simulink model "SF035A_DampgPahFwl"  (R2013b)
settings: Solver=FixedStepDiscrete  SolverMode=SingleTasking  StartTime=0.0  StopTime=1  FixedStep=0.002  RelTol=1e-3
undefined symbols (not defined in the file): ARCHGLBPRM_2MILLISEC_SEC_F32, DampgPahFwlDampgCmdFwlOverLimDiagcFailStep, DampgPahFwlDampgCmdFwlOverLimDiagcPassStep, DampgPahFwlInertiaCmpCmdFwlOverLimDiagcFailStep, DampgPahFwlInertiaCmpCmdFwlOverLimDiagcPassStep, DMPGCMDREACHED_CNT_U08, MfgEnaSt1, NtcNr1, NtcSts1, sigbuilder_block, SigQlfr1, VBICCMDREACHED_CNT_U08
libraries: simulink x23, Fil x12, FixdToFloat x7, FloatToFixd x5, BilnrIntrpnCmnX x4, LnrIntrpn x3, NxtrLim x3, NxtrAbslt x2, NxtrSign x2, NxtrMax x1
(part 1 of 3)
settings Model: Creator=HariP  LastModifiedBy=SNEHAP1
settings SolverCC: AutoInsertRateTranBlk=on  InsertRTBMode=Always
settings DataIOCC: LimitDataPoints=off  SaveFormat=Structure  ReturnWorkspaceOutputs=on
settings OptimizationCC: BlockReduction=off  InlineParams=on  ZeroExternalMemoryAtStartup=off  ZeroInternalMemoryAtStartup=off  OptimizeModelRefInitCode=on  LifeSpan=1
settings DebuggingCC: SignalInfNanChecking=error  SignalRangeChecking=warning  UnderspecifiedInitializationDetection=Simplified  SolverPrmCheckMsg=error  InheritedTsInSrcMsg=error  DiscreteInheritContinuousMsg=error  SingleTaskRateTransMsg=error  TasksWithSamePriorityMsg=error  SigSpecEnsureSampleTimeMsg=error  CheckMatrixSingularityMsg=error  ParameterUnderflowMsg=error  ParameterPrecisionLossMsg=error  ParameterTunabilityLossMsg=error  FixptConstUnderflowMsg=warning  FixptConstOverflowMsg=warning  VectorMatrixConversionMsg=error  SignalLabelMismatchMsg=error  UnconnectedInputMsg=error  UnconnectedOutputMsg=error  UnconnectedLineMsg=error  SFcnCompatibilityMsg=error  UniqueDataStoreMsg=warning  BusObjectLabelMismatch=error  RootOutportRequireBusObject=error  AssertControl=DisableAll  ModelReferenceIOMsg=error  ModelReferenceVersionMismatchMessage=warning  ModelReferenceIOMismatchMessage=error  ModelReferenceCSMismatchMessage=warning  ModelReferenceDataLoggingMessage=error  StateNameClashWarn=warning  StrictBusMsg=ErrorOnBusTreatedAsVector  NonBusSignalsTreatedAsBus=error  SFUnexpectedBacktrackingDiag=error  SFInvalidInputDataAccessInChartInitDiag=error  SFNoUnconditionalDefaultTransitionDiag=error  SFTransitionOutsideNaturalParentDiag=error  SFUnconditionalTransitionShadowingDiag=error  SFUndirectedBroadcastEventsDiag=error
settings ModelReferenceCC: ModelReferenceNumInstancesAllowed=Single
settings RTWCC: SystemTargetFile=autosar.tlc  GenCodeOnly=on  TemplateMakefile=ert_default_tmf  Description=AUTOSAR  GenerateReport=on  ProcessScript=autosar_make_rtw_hook  LaunchReport=on
settings CodeAppCC: GenerateComments=off  IgnoreCustomStorageClasses=off  CustomSymbolStrType=$N$R$M  CustomSymbolStrBlkIO=$N$M  SimulinkBlockComments=off
settings STFCustomTargetCC: ParMdlRefBuildCompliant=on  CompOptLevelCompliant=on  IncludeMdlTerminateFcn=off  CombineOutputUpdateFcns=on  SuppressErrorStatus=on  ERTFirstTimeCompliant=on  ERTCustomFileBanners=on  SupportNonFinite=off  SupportComplex=off  SupportContinuousTime=off  SupportNonInlinedSFcns=off  MATLABClassNameForMDSCustomization=Simulink.SoftwareTarget.ERTCustomization  AutosarCompliant=on  GRTInterface=off  SystemTargetFile=autosar.tlc
settings ERTTargetCC: CodeReplacementLibrary=ANSI_C  ConcurrentExecutionCompliant=off  IncludeMdlTerminateFcn=off  SuppressErrorStatus=on  SupportNonFinite=off  SupportComplex=off  ModelStepFunctionPrototypeControlCompliant=off  CPPClassGenCompliant=off  AutosarCompliant=on  InlinedParameterPlacement=NonHierarchical  ERTCustomFileTemplate=example_file_process.tlc  EnableUserReplacementTypes=on

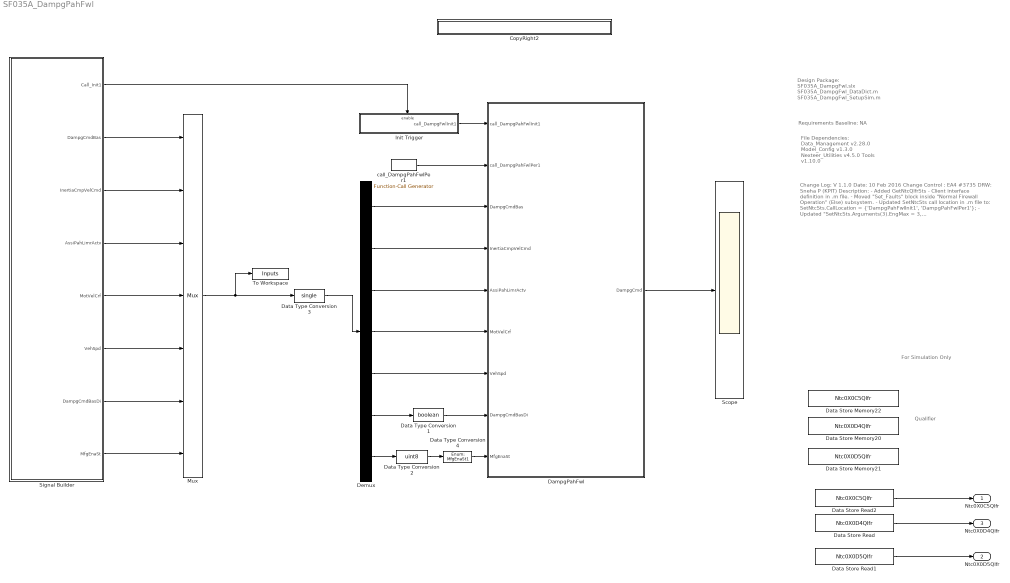
== system SF035A_DampgPahFwl ==
  note: Qualifier
  note: For Simulation Only
  note: Requirements Baseline: NA
  note: Design Package:
      | SF035A_DampgFwl.slx
      | SF035A_DampgFwl_DataDict.m
      | SF035A_DampgFwl_SetupSim.m
  note: File Dependencies:
      | Data_Management v2.28.0
      | Model_Config v1.3.0
      | Nexteer_Utilities v4.5.0
      | Tools v1.10.0
  note: Change Log:  V 1.1.0
      | Date: 10 Feb 2016
      | Change Control :  EA4 #3735
      | DRW: Sneha P (KPIT)
      | Description:
      | - Added GetNtcQlfrSts - Client interface definition in .m file.
      | - Moved "Set_Faults" block inside "Normal Firewall Operation"
      |   (Else) subsystem.
      | - Updated SetNtcSts call location in .m file to:
      |   SetNtcSts.CallLocation = {'DampgPahFwlInit1', 'DampgPahFwlPer1'};
      | - Updated "SetNtcSts.Arguments(3).EngMax = 3,
      |   SetNtcSts.Arguments(3).EngDT = enum.NtcSts1;,
      |   SetNtcSts.Arguments(3).Units = 'Cnt' in .m file.
      |
      |
      | Change Log:  V 1.0.0
      | Date: 01 Feb 2016
      | Change Control #:  EA4 #3606
      | DRW: Hari Prasad / Muragesh Asundi (KPIT)
      | Description:
      | - Initial Release of EA4 V1.0.0 from EA3 V12.0.X
  CopyRight2 : Subsystem  Description=|  mask(Copyright Information){none=on}
      | Copyright info block.                                               
      |                                                                     
      | Place copyright information at the top of every subsystem in design.
      mask prompts: none "No parameters"
      mask help: Place copyright information at the top of every subsystem in design.
      mask Display:
      | NxtrConf = 'Nexteer Confidential';
      | 
      | sys = bdroot; %handle for the current model ("system")
      | first = get_param(sys,'Created');
      | first = first(end-3:end);  %year is last four digits
      | 
      | last = get_param(sys,'LastModifiedDate');
      | if isempty(last)
      |     last = datestr(now,'yyyy');
      | else
      |     last = last(end-3:end);
      | end
      | 
      | if strcmp(first,last)
      |     fprintf('%s -- Copyright %s Nexteer',NxtrConf,first)
      | else
      |     fprintf('%s -- %s%s- %s Nexteer',NxtrConf,char(169),first,last)
      | end
  DampgPahFwl : Subsystem
  Data Store Memory20 : DataStoreMemory  DataStoreName=Ntc0X0D4Qlfr  InitialValue=SigQlfr1.SIGQLFR_NORES  OutDataTypeStr=Enum: SigQlfr1
  Data Store Memory21 : DataStoreMemory  DataStoreName=Ntc0X0D5Qlfr  InitialValue=SigQlfr1.SIGQLFR_NORES  OutDataTypeStr=Enum: SigQlfr1
  Data Store Memory22 : DataStoreMemory  DataStoreName=Ntc0X0C5Qlfr  InitialValue=SigQlfr1.SIGQLFR_NORES  OutDataTypeStr=Enum: SigQlfr1
  Data Store Read : DataStoreRead  DataStoreName=Ntc0X0D4Qlfr  SampleTime=0.002
  Data Store Read1 : DataStoreRead  DataStoreName=Ntc0X0D5Qlfr  SampleTime=0.002
  Data Store Read2 : DataStoreRead  DataStoreName=Ntc0X0C5Qlfr  SampleTime=0.002
  Data Type Conversion1 : DataTypeConversion  OutDataTypeStr=boolean
  Data Type Conversion2 : DataTypeConversion  OutDataTypeStr=uint8
  Data Type Conversion3 : DataTypeConversion  OutDataTypeStr=single
  Data Type Conversion4 : DataTypeConversion  OutDataTypeStr=Enum: MfgEnaSt1
  Demux : Demux  Outputs=7
  Init Trigger : Subsystem  TreatAsAtomicUnit=on
  Mux : Mux  Inputs=7
  Scope : Scope
  Signal Builder : Subsystem  Tag=STV Subsys  LoadFcn=sigbuilder_block('load');  StartFcn=sigbuilder_block('start');  StopFcn=sigbuilder_block('stop');  ClipboardFcn=sigbuilder_block('clipboard');  mask(Sigbuilder block){}
      mask help: Simulink:masks:SigbuilderBlock_MD
      mask init:
      | if ~strcmp(get_param(bdroot(gcbh),'SimulationStatus'),'stopped') tuvar = sigbuilder_block('maskInit'); end
      settings: CopyFcn=sigbuilder_block('copy');  DeleteFcn=sigbuilder_block('delete');  ModelCloseFcn=sigbuilder_block('modelClose');  PreSaveFcn=sigbuilder_block('preSave');  PauseFcn=sigbuilder_block('pause');  ContinueFcn=sigbuilder_block('continue');  NameChangeFcn=sigbuilder_block('namechange');  OpenFcn=sigbuilder_block('open',[0 30 1024.5 489 ]);  CloseFcn=sigbuilder_block('close');
      mask Display: plot(0, 0, 100, 100,[2, 2, 32, 32, 2], [68, 8, 8, 68, 68],[32, 2], [38, 38], [32, 19, 2],[53, 60, 44], [32, 17, 17, 2],[16, 16, 31, 31]);txt = getActiveGroup(gcbh);text(2, 100, txt,'verticalAlignment', 'top');
  To Workspace : ToWorkspace  VariableName=Inputs  SampleTime=-1
  call_DampgPahFwlPer1 : simulink/Ports & Subsystems/Function-Call Generator  RequirementInfo={} %GIDa_4a149a05_295f_452b_ba1c_52fd600be539  sample_time=0.002  numberOfIterations=1
  Ntc0X0C5Qlfr : Outport
  Ntc0X0D5Qlfr : Outport  Port=2
  Ntc0X0D4Qlfr : Outport  Port=3
  wires:
  DampgPahFwl/1(DampgCmd) -> Scope/1
  Init Trigger/1(call_DampgFwlInit1) -> DampgPahFwl/1(call_DampgPahFwlInit1)
  call_DampgPahFwlPer1/1 -> DampgPahFwl/2(call_DampgPahFwlPer1)
  Data Store Read/1 -> Ntc0X0D4Qlfr/1
  Data Store Read1/1 -> Ntc0X0D5Qlfr/1
  Data Store Read2/1 -> Ntc0X0C5Qlfr/1
  Mux/1 -> To Workspace/1, Data Type Conversion3/1
  Data Type Conversion3/1 -> Demux/1
  Demux/4 -> DampgPahFwl/6(MotVelCrf)
  Demux/2 -> DampgPahFwl/4(InertiaCmpVelCmd)
  Demux/5 -> DampgPahFwl/7(VehSpd)
  Demux/1 -> DampgPahFwl/3(DampgCmdBas)
  Demux/6 -> Data Type Conversion1/1
  Demux/7 -> Data Type Conversion2/1
  Signal Builder/1(Call_Init1) -> Init Trigger/Enable
  Signal Builder/4(AssiPahLimrActv) -> Mux/3
  Signal Builder/5(MotVelCrf) -> Mux/4
  Signal Builder/3(InertiaCmpVelCmd) -> Mux/2
  Signal Builder/6(VehSpd) -> Mux/5
  Signal Builder/2(DampgCmdBas) -> Mux/1
  Signal Builder/7(DampgCmdBasDi) -> Mux/6
  Signal Builder/8(MfgEnaSt) -> Mux/7
  Data Type Conversion1/1 -> DampgPahFwl/8(DampgCmdBasDi)
  Demux/3 -> DampgPahFwl/5(AssiPahLimrActv)
  Data Type Conversion2/1 -> Data Type Conversion4/1
  Data Type Conversion4/1 -> DampgPahFwl/9(MfgEnaSt)

== system SF035A_DampgPahFwl/CopyRight2 ==

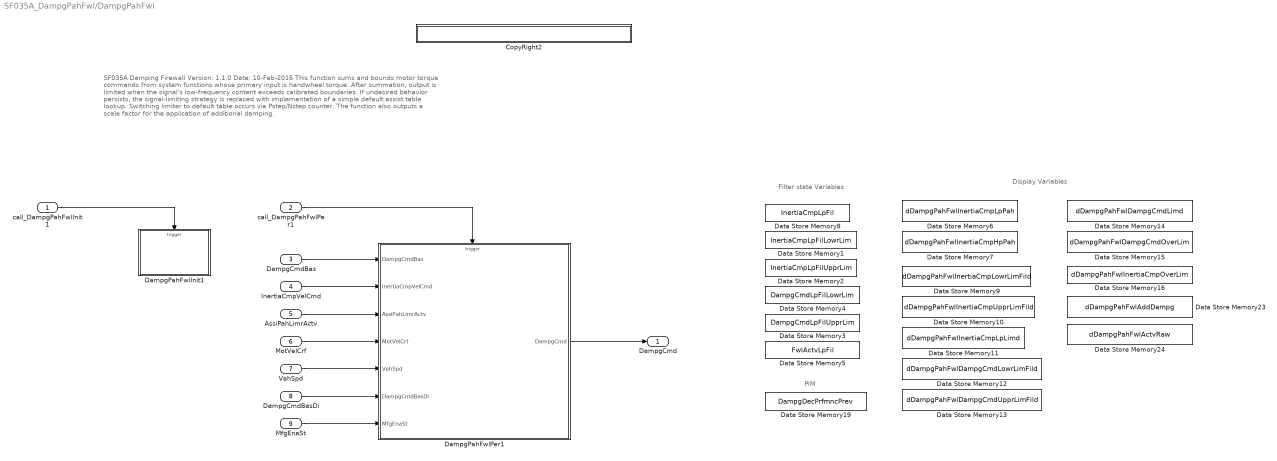
== system SF035A_DampgPahFwl/DampgPahFwl ==
  note: PIM
  note: Filter state Variables
  note: Display Variables
  note: SF035A Damping Firewall
      | Version: 1.1.0      Date: 10-Feb-2016
      |
      | This function sums and bounds motor torque commands from system functions whose primary input is handwheel torque.  After summation, output is limited when the signal's low-frequency content
      | exceeds calibrated boundaries.  If undesired behavior persists,  the signal-limiting strategy is replaced with implementation of a simple default assist table lookup.  Switching limiter to default table
      | occurs via Pstep/Nstep counter.  The function also outputs a scale factor for the application of additional damping.
  call_DampgPahFwlInit1 : Inport
  call_DampgPahFwlPer1 : Inport  Port=2
  DampgCmdBas : Inport  Port=3
  InertiaCmpVelCmd : Inport  Port=4
  AssiPahLimrActv : Inport  Port=5
  MotVelCrf : Inport  Port=6
  VehSpd : Inport  Port=7
  DampgCmdBasDi : Inport  Port=8
  MfgEnaSt : Inport  Port=9
  CopyRight2 : Subsystem  Description=|  mask(Copyright Information){none=on}
      | Copyright info block.                                               
      |                                                                     
      | Place copyright information at the top of every subsystem in design.
      mask prompts: none "No parameters"
      mask help: Place copyright information at the top of every subsystem in design.
      mask Display:
      | NxtrConf = 'Nexteer Confidential';
      | 
      | sys = bdroot; %handle for the current model ("system")
      | first = get_param(sys,'Created');
      | first = first(end-3:end);  %year is last four digits
      | 
      | last = get_param(sys,'LastModifiedDate');
      | if isempty(last)
      |     last = datestr(now,'yyyy');
      | else
      |     last = last(end-3:end);
      | end
      | 
      | if strcmp(first,last)
      |     fprintf('%s -- Copyright %s Nexteer',NxtrConf,first)
      | else
      |     fprintf('%s -- %s%s- %s Nexteer',NxtrConf,char(169),first,last)
      | end
  DampgPahFwlInit1 : Subsystem  TreatAsAtomicUnit=on
  DampgPahFwlPer1 : Subsystem
  Data Store Memory1 : DataStoreMemory  DataStoreName=InertiaCmpLpFilLowrLim  InitialValue=struct('FilSt',single(0),'FilGain',single(0))  OutDataTypeStr=Bus: FilLpRec1  StateMustResolveToSignalObject=on
  Data Store Memory10 : DataStoreMemory  DataStoreName=dDampgPahFwlInertiaCmpUpprLimFild  StateMustResolveToSignalObject=on
  Data Store Memory11 : DataStoreMemory  DataStoreName=dDampgPahFwlInertiaCmpLpLimd  InitialValue=[]  StateMustResolveToSignalObject=on
  Data Store Memory12 : DataStoreMemory  DataStoreName=dDampgPahFwlDampgCmdLowrLimFild  InitialValue=[]  StateMustResolveToSignalObject=on
  Data Store Memory13 : DataStoreMemory  DataStoreName=dDampgPahFwlDampgCmdUpprLimFild  InitialValue=[]  StateMustResolveToSignalObject=on
  Data Store Memory14 : DataStoreMemory  DataStoreName=dDampgPahFwlDampgCmdLimd  InitialValue=[]  StateMustResolveToSignalObject=on
  Data Store Memory15 : DataStoreMemory  DataStoreName=dDampgPahFwlDampgCmdOverLim  InitialValue=[]  StateMustResolveToSignalObject=on
  Data Store Memory16 : DataStoreMemory  DataStoreName=dDampgPahFwlInertiaCmpOverLim  InitialValue=[]  StateMustResolveToSignalObject=on
  Data Store Memory19 : DataStoreMemory  DataStoreName=DampgDecPrfmncPrev  StateMustResolveToSignalObject=on
  Data Store Memory2 : DataStoreMemory  DataStoreName=InertiaCmpLpFilUpprLim  InitialValue=struct('FilSt',single(0),'FilGain',single(0))  OutDataTypeStr=Bus: FilLpRec1  StateMustResolveToSignalObject=on
  Data Store Memory23 : DataStoreMemory  DataStoreName=dDampgPahFwlAddDampg  InitialValue=[]  StateMustResolveToSignalObject=on
  Data Store Memory24 : DataStoreMemory  DataStoreName=dDampgPahFwlActvRaw  InitialValue=[]  StateMustResolveToSignalObject=on
  Data Store Memory3 : DataStoreMemory  DataStoreName=DampgCmdLpFilUpprLim  InitialValue=struct('FilSt',single(0),'FilGain',single(0))  OutDataTypeStr=Bus: FilLpRec1  StateMustResolveToSignalObject=on
  Data Store Memory4 : DataStoreMemory  DataStoreName=DampgCmdLpFilLowrLim  InitialValue=struct('FilSt',single(0),'FilGain',single(0))  OutDataTypeStr=Bus: FilLpRec1  StateMustResolveToSignalObject=on
  Data Store Memory5 : DataStoreMemory  DataStoreName=FwlActvLpFil  InitialValue=struct('FilSt',single(0),'FilGain',single(0))  OutDataTypeStr=Bus: FilLpRec1  StateMustResolveToSignalObject=on
  Data Store Memory6 : DataStoreMemory  DataStoreName=dDampgPahFwlInertiaCmpLpPah  InitialValue=[]  StateMustResolveToSignalObject=on
  Data Store Memory7 : DataStoreMemory  DataStoreName=dDampgPahFwlInertiaCmpHpPah  InitialValue=[]  StateMustResolveToSignalObject=on
  Data Store Memory8 : DataStoreMemory  DataStoreName=InertiaCmpLpFil  InitialValue=struct('FilSt',single(0),'FilGain',single(0))  OutDataTypeStr=Bus: FilLpRec1  StateMustResolveToSignalObject=on
  Data Store Memory9 : DataStoreMemory  DataStoreName=dDampgPahFwlInertiaCmpLowrLimFild  InitialValue=[]  StateMustResolveToSignalObject=on
  DampgCmd : Outport
  wires:
  DampgPahFwlPer1/1(DampgCmd) -> DampgCmd/1
  call_DampgPahFwlPer1/1 -> DampgPahFwlPer1/Trigger
  DampgCmdBas/1 -> DampgPahFwlPer1/1(DampgCmdBas)
  InertiaCmpVelCmd/1 -> DampgPahFwlPer1/2(InertiaCmpVelCmd)
  AssiPahLimrActv/1 -> DampgPahFwlPer1/3(AssiPahLimrActv)
  VehSpd/1 -> DampgPahFwlPer1/5(VehSpd)
  MotVelCrf/1 -> DampgPahFwlPer1/4(MotVelCrf)
  DampgCmdBasDi/1 -> DampgPahFwlPer1/6(DampgCmdBasDi)
  MfgEnaSt/1 -> DampgPahFwlPer1/7(MfgEnaSt)
  call_DampgPahFwlInit1/1 -> DampgPahFwlInit1/Trigger

== system SF035A_DampgPahFwl/Init Trigger ==
  Enable : EnablePort
  CopyRight2 : Subsystem  Description=|  mask(Copyright Information){none=on}
      | Copyright info block.                                               
      |                                                                     
      | Place copyright information at the top of every subsystem in design.
      mask prompts: none "No parameters"
      mask help: Place copyright information at the top of every subsystem in design.
      mask Display:
      | NxtrConf = 'Nexteer Confidential';
      | 
      | sys = bdroot; %handle for the current model ("system")
      | first = get_param(sys,'Created');
      | first = first(end-3:end);  %year is last four digits
      | 
      | last = get_param(sys,'LastModifiedDate');
      | if isempty(last)
      |     last = datestr(now,'yyyy');
      | else
      |     last = last(end-3:end);
      | end
      | 
      | if strcmp(first,last)
      |     fprintf('%s -- Copyright %s Nexteer',NxtrConf,first)
      | else
      |     fprintf('%s -- %s%s- %s Nexteer',NxtrConf,char(169),first,last)
      | end
  call_DampgPahFwlInit : simulink/Ports & Subsystems/Function-Call Generator  sample_time=0  numberOfIterations=1
  call_DampgFwlInit1 : Outport
  wires:
  call_DampgPahFwlInit/1 -> call_DampgFwlInit1/1

== system SF035A_DampgPahFwl/Signal Builder ==
  Demux : Demux  Tag=STV Demux  Outputs=8
  FromWs : FromWorkspace  Tag=STV FromWs  VariableName=tuvar  SampleTime=0
      SigBuilderData=|
      | common.afterFinalStr = 'Extrapolate'
      | common.sampleTime = 0
      | dataSet.timeRange = [0 0.31]
      | dataSet.name = 'TestCase_1'
      | sbobj.Name = 'Signal Builder'
      | sbobj.Groups.Name = 'TestCase_1'
      | sbobj.Groups.Signals(1).Name = 'Call_Init1'
      | sbobj.Groups.Signals(1).XData = [0 0.002 0.004 0.006 0.008 0.01 0.012 0.014 0.016 0.018 0.02 0.022 0.024 0.026 0.028 0.03 0.032 0.034 0.036 0.038 0.04 0.042 0.044 0.046 0.048 0.05 0.052 0.054 0.056 0.058 0.06 0.062 0.064 0.066 0.068 0.07 0.072 0.074 0.076 0.078 0.08 0.082 0.084 0.086 0.088 0.09 0.092 0.094 0.096 0.098 0.1 0.102 0.104 0.106 0.108 0.11 0.112 0.114 0.116 0.118 0.12 0.122 0.124 0.126 0.128 0.13 0.132 0.134 0.136 0.138 0.14 0.142 0.144 0.146 0.148 0.15 0.152 0.154 0.156 0.158 0.16 0.162 0.164 0.166 0.168 0.17 0.172 0.174 0.176 0.178 0.18 0.182 0.184 0.186 0.188 0.19 0.192 0.194 0.196 0.198 0.2 0.202 0.204 0.206 0.208 0.21 0.212 0.214 0.216 0.218 0.22 0.222 0.224 0.226 0.228 0.23 0.232 0.234 0.236 0.238 0.24 0.242 0.244 0.246 0.248 0.25 0.252 0.254 0.256 0.258 0.26 0.262 0.264 0.266 0.268 0.27 0.272 0.274 0.276 0.278 0.28 0.282 0.284 0.286 0.288 0.29 0.292 0.294 0.296 0.298 0.3 0.302 0.304 0.306 0.308 0.31]
      | sbobj.Groups.Signals(1).YData = [1 0 0 0 0 0 0 0 0 0 0 0 0 0 0 0 0 0 0 0 0 0 0 0 0 0 0 0 0 0 0 0 0 0 0 0 0 0 0 0 0 0 0 0 0 0 0 0 0 0 0 0 0 0 0 0 0 0 0 0 0 0 0 0 0 0 0 0 0 0 0 0 0 0 0 0 0 0 0 0 0 0 0 0 0 0 0 0 0 0 0 0 0 0 0 0 0 0 0 0 0 0 0 0 0 0 0 0 0 0 0 0 0 0 0 0 0 0 0 0 0 0 0 0 0 0 0 0 0 0 0 0 0 0 0 0 0 0 0 0 0 0 0 0 0 0 0 0 0 0 0 0 0 0 0 0]
      | sbobj.Groups.Signals(2).Name = 'DampgCmdBas'
      | sbobj.Groups.Signals(2).XData = [0 0.002 0.004 0.006 0.008 0.01 0.012 0.014 0.016 0.018 0.02 0.022 0.024 0.026 0.028 0.03 0.032 0.034 0.036 0.038 0.04 0.042 0.044 0.046 0.048 0.05 0.052 0.054 0.056 0.058 0.06 0.062 0.064 0.066 0.068 0.07 0.072 0.074 0.076 0.078 0.08 0.082 0.084 0.086 0.088 0.09 0.092 0.094 0.096 0.098 0.1 0.102 0.104 0.106 0.108 0.11 0.112 0.114 0.116 0.118 0.12 0.122 0.124 0.126 0.128 0.13 0.132 0.134 0.136 0.138 0.14 0.142 0.144 0.146 0.148 0.15 0.152 0.154 0.156 0.158 0.16 0.162 0.164 0.166 0.168 0.17 0.172 0.174 0.176 0.178 0.18 0.182 0.184 0.186 0.188 0.19 0.192 0.194 0.196 0.198 0.2 0.202 0.204 0.206 0.208 0.21 0.212 0.214 0.216 0.218 0.22 0.222 0.224 0.226 0.228 0.23 0.232 0.234 0.236 0.238 0.24 0.242 0.244 0.246 0.248 0.25 0.252 0.254 0.256 0.258 0.26 0.262 0.264 0.266 0.268 0.27 0.272 0.274 0.276 0.278 0.28 0.282 0.284 0.286 0.288 0.29 0.292 0.294 0.296 0.298 0.3 0.302 0.304 0.306 0.308 0.31]
      | sbobj.Groups.Signals(2).YData = [-8.8 -8.78263521017 -8.70559653007 -8.56749434528 -8.3692973434 -8.11239573398 -7.79859149723 -7.43008574442 -7.00946327861 -6.5396744642 -6.02401453217 -5.46610046645 ... (156 elements, 1x156)]
      | sbobj.Groups.Signals(3).Name = 'InertiaCmpVelCmd'
      | sbobj.Groups.Signals(3).XData = [0 0.002 0.004 0.006 0.008 0.01 0.012 0.014 0.016 0.018 0.02 0.022 0.024 0.026 0.028 0.03 0.032 0.034 0.036 0.038 0.04 0.042 0.044 0.046 0.048 0.05 0.052 0.054 0.056 0.058 0.06 0.062 0.064 0.066 0.068 0.07 0.072 0.074 0.076 0.078 0.08 0.082 0.084 0.086 0.088 0.09 0.092 0.094 0.096 0.098 0.1 0.102 0.104 0.106 0.108 0.11 0.112 0.114 0.116 0.118 0.12 0.122 0.124 0.126 0.128 0.13 0.132 0.134 0.136 0.138 0.14 0.142 0.144 0.146 0.148 0.15 0.152 0.154 0.156 0.158 0.16 0.162 0.164 0.166 0.168 0.17 0.172 0.174 0.176 0.178 0.18 0.182 0.184 0.186 0.188 0.19 0.192 0.194 0.196 0.198 0.2 0.202 0.204 0.206 0.208 0.21 0.212 0.214 0.216 0.218 0.22 0.222 0.224 0.226 0.228 0.23 0.232 0.234 0.236 0.238 0.24 0.242 0.244 0.246 0.248 0.25 0.252 0.254 0.256 0.258 0.26 0.262 0.264 0.266 0.268 0.27 0.272 0.274 0.276 0.278 0.28 0.282 0.284 0.286 0.288 0.29 0.292 0.294 0.296 0.298 0.3 0.302 0.304 0.306 0.308 0.31]
      | sbobj.Groups.Signals(3).YData = [0 0.736365021324 1.4675649711 2.18847100705 2.8940264913 3.57928245907 4.2394323321 4.86984563334 5.46610046645 6.02401453217 6.5396744642 7.00946327861 ... (156 elements, 1x156)]
      | sbobj.Groups.Signals(4).Name = 'AssiPahLimrActv'
      | sbobj.Groups.Signals(4).XData = [0 0.002 0.004 0.006 0.008 0.01 0.012 0.014 0.016 0.018 0.02 0.022 0.024 0.026 0.028 0.03 0.032 0.034 0.036 0.038 0.04 0.042 0.044 0.046 0.048 0.05 0.052 0.054 0.056 0.058 0.06 0.062 0.064 0.066 0.068 0.07 0.072 0.074 0.076 0.078 0.08 0.082 0.084 0.086 0.088 0.09 0.092 0.094 0.096 0.098 0.1 0.102 0.104 0.106 0.108 0.11 0.112 0.114 0.116 0.118 0.12 0.122 0.124 0.126 0.128 0.13 0.132 0.134 0.136 0.138 0.14 0.142 0.144 0.146 0.148 0.15 0.152 0.154 0.156 0.158 0.16 0.162 0.164 0.166 0.168 0.17 0.172 0.174 0.176 0.178 0.18 0.182 0.184 0.186 0.188 0.19 0.192 0.194 0.196 0.198 0.2 0.202 0.204 0.206 0.208 0.21 0.212 0.214 0.216 0.218 0.22 0.222 0.224 0.226 0.228 0.23 0.232 0.234 0.236 0.238 0.24 0.242 0.244 0.246 0.248 0.25 0.252 0.254 0.256 0.258 0.26 0.262 0.264 0.266 0.268 0.27 0.272 0.274 0.276 0.278 0.28 0.282 0.284 0.286 0.288 0.29 0.292 0.294 0.296 0.298 0.3 0.302 0.304 0.306 0.308 0.31]
      | sbobj.Groups.Signals(4).YData = [0 0 0 0 0 0 0 0 0 0 0 0 0 0 0 0 0 0 0 0 0 0 0 0 0 0 0 0 0 0 0 0 0 0 0 0 0 0 0 0 0 0 0 0 0 0 0 0 0 0 0 0 0 0 0 0 0 1 1 1 1 1 1 1 1 1 1 1 1 1 1 1 1 1 1 1 1 1 1 1 1 1 1 1 1 1 1 1 1 1 1 1 1 1 1 1 1 1 1 1 1 1 1 1 1 1 1 1 1 1 1 1 1 1 1 1 1 1 1 1 1 1 1 1 1 1 1 1 1 1 1 1 1 1 1 1 1 1 1 1 1 1 1 1 1 1 1 1 1 1 1 1 1 1 1 1]
      | sbobj.Groups.Signals(5).Name = 'MotVelCrf'
      | sbobj.Groups.Signals(5).XData = [0 0.002 0.004 0.006 0.008 0.01 0.012 0.014 0.016 0.018 0.02 0.022 0.024 0.026 0.028 0.03 0.032 0.034 0.036 0.038 0.04 0.042 0.044 0.046 0.048 0.05 0.052 0.054 0.056 0.058 0.06 0.062 0.064 0.066 0.068 0.07 0.072 0.074 0.076 0.078 0.08 0.082 0.084 0.086 0.088 0.09 0.092 0.094 0.096 0.098 0.1 0.102 0.104 0.106 0.108 0.11 0.112 0.114 0.116 0.118 0.12 0.122 0.124 0.126 0.128 0.13 0.132 0.134 0.136 0.138 0.14 0.142 0.144 0.146 0.148 0.15 0.152 0.154 0.156 0.158 0.16 0.162 0.164 0.166 0.168 0.17 0.172 0.174 0.176 0.178 0.18 0.182 0.184 0.186 0.188 0.19 0.192 0.194 0.196 0.198 0.2 0.202 0.204 0.206 0.208 0.21 0.212 0.214 0.216 0.218 0.22 0.222 0.224 0.226 0.228 0.23 0.232 0.234 0.236 0.238 0.24 0.242 0.244 0.246 0.248 0.25 0.252 0.254 0.256 0.258 0.26 0.262 0.264 0.266 0.268 0.27 0.272 0.274 0.276 0.278 0.28 0.282 0.284 0.286 0.288 0.29 0.292 0.294 0.296 0.298 0.3 0.302 0.304 0.306 0.308 0.31]
      | sbobj.Groups.Signals(5).YData = [0 278.03529385 538.600607646 765.323664428 943.958620711 1063.28118522 1115.79388238 1098.19714631 1011.59664466 861.433805423 657.143912063 411.563249901 ... (156 elements, 1x156)]
      | sbobj.Groups.Signals(6).Name = 'VehSpd'
      | sbobj.Groups.Signals(6).XData = [0 0.002 0.004 0.006 0.008 0.01 0.012 0.014 0.016 0.018 0.02 0.022 0.024 0.026 0.028 0.03 0.032 0.034 0.036 0.038 0.04 0.042 0.044 0.046 0.048 0.05 0.052 0.054 0.056 0.058 0.06 0.062 0.064 0.066 0.068 0.07 0.072 0.074 0.076 0.078 0.08 0.082 0.084 0.086 0.088 0.09 0.092 0.094 0.096 0.098 0.1 0.102 0.104 0.106 0.108 0.11 0.112 0.114 0.116 0.118 0.12 0.122 0.124 0.126 0.128 0.13 0.132 0.134 0.136 0.138 0.14 0.142 0.144 0.146 0.148 0.15 0.152 0.154 0.156 0.158 0.16 0.162 0.164 0.166 0.168 0.17 0.172 0.174 0.176 0.178 0.18 0.182 0.184 0.186 0.188 0.19 0.192 0.194 0.196 0.198 0.2 0.202 0.204 0.206 0.208 0.21 0.212 0.214 0.216 0.218 0.22 0.222 0.224 0.226 0.228 0.23 0.232 0.234 0.236 0.238 0.24 0.242 0.244 0.246 0.248 0.25 0.252 0.254 0.256 0.258 0.26 0.262 0.264 0.266 0.268 0.27 0.272 0.274 0.276 0.278 0.28 0.282 0.284 0.286 0.288 0.29 0.292 0.294 0.296 0.298 0.3 0.302 0.304 0.306 0.308 0.31]
      | sbobj.Groups.Signals(6).YData = [0 21.3984590556 42.7593779428 64.0452823514 85.2188295719 106.242874008 127.080532341 147.695248239 168.050856483 188.111646422 207.842424612 227.208576563 ... (156 elements, 1x156)]
      | sbobj.Groups.Signals(7).Name = 'DampgCmdBasDi'
      | sbobj.Groups.Signals(7).XData = [0 0.002 0.004 0.006 0.008 0.01 0.012 0.014 0.016 0.018 0.02 0.022 0.024 0.026 0.028 0.03 0.032 0.034 0.036 0.038 0.04 0.042 0.044 0.046 0.048 0.05 0.052 0.054 0.056 0.058 0.06 0.062 0.064 0.066 0.068 0.07 0.072 0.074 0.076 0.078 0.08 0.082 0.084 0.086 0.088 0.09 0.092 0.094 0.096 0.098 0.1 0.102 0.104 0.106 0.108 0.11 0.112 0.114 0.116 0.118 0.12 0.122 0.124 0.126 0.128 0.13 0.132 0.134 0.136 0.138 0.14 0.142 0.144 0.146 0.148 0.15 0.152 0.154 0.156 0.158 0.16 0.162 0.164 0.166 0.168 0.17 0.172 0.174 0.176 0.178 0.18 0.182 0.184 0.186 0.188 0.19 0.192 0.194 0.196 0.198 0.2 0.202 0.204 0.206 0.208 0.21 0.212 0.214 0.216 0.218 0.22 0.222 0.224 0.226 0.228 0.23 0.232 0.234 0.236 0.238 0.24 0.242 0.244 0.246 0.248 0.25 0.252 0.254 0.256 0.258 0.26 0.262 0.264 0.266 0.268 0.27 0.272 0.274 0.276 0.278 0.28 0.282 0.284 0.286 0.288 0.29 0.292 0.294 0.296 0.298 0.3 0.302 0.304 0.306 0.308 0.31]
      | sbobj.Groups.Signals(7).YData = [0 0 0 0 0 0 0 0 0 0 0 0 0 0 0 0 0 0 0 0 0 0 0 0 0 0 0 0 0 0 0 0 0 0 0 0 0 0 0 0 0 0 0 0 0 0 0 0 0 0 0 0 0 0 0 0 0 0 0 0 0 0 0 0 0 0 0 0 0 0 0 0 0 0 0 0 1 1 1 1 1 1 1 1 1 1 1 1 1 1 1 1 1 1 1 1 1 1 1 1 1 1 1 1 1 1 1 1 1 1 1 1 1 1 1 1 1 1 1 1 1 1 1 1 1 1 1 1 1 1 1 1 1 1 1 1 1 1 1 1 1 1 1 1 1 1 1 1 1 1 1 1 1 1 1 1]
      | sbobj.Groups.Signals(8).Name = 'MfgEnaSt'
      | sbobj.Groups.Signals(8).XData = [0 0.002 0.004 0.006 0.008 0.01 0.012 0.014 0.016 0.018 0.02 0.022 0.024 0.026 0.028 0.03 0.032 0.034 0.036 0.038 0.04 0.042 0.044 0.046 0.048 0.05 0.052 0.054 0.056 0.058 0.06 0.062 0.064 0.066 0.068 0.07 0.072 0.074 0.076 0.078 0.08 0.082 0.084 0.086 0.088 0.09 0.092 0.094 0.096 0.098 0.1 0.102 0.104 0.106 0.108 0.11 0.112 0.114 0.116 0.118 0.12 0.122 0.124 0.126 0.128 0.13 0.132 0.134 0.136 0.138 0.14 0.142 0.144 0.146 0.148 0.15 0.152 0.154 0.156 0.158 0.16 0.162 0.164 0.166 0.168 0.17 0.172 0.174 0.176 0.178 0.18 0.182 0.184 0.186 0.188 0.19 0.192 0.194 0.196 0.198 0.2 0.202 0.204 0.206 0.208 0.21 0.212 0.214 0.216 0.218 0.22 0.222 0.224 0.226 0.228 0.23 0.232 0.234 0.236 0.238 0.24 0.242 0.244 0.246 0.248 0.25 0.252 0.254 0.256 0.258 0.26 0.262 0.264 0.266 0.268 0.27 0.272 0.274 0.276 0.278 0.28 0.282 0.284 0.286 0.288 0.29 0.292 0.294 0.296 0.298 0.3 0.302 0.304 0.306 0.308 0.31]
      | sbobj.Groups.Signals(8).YData = [2 2 2 2 2 2 2 2 2 2 2 2 2 2 2 2 2 2 2 2 2 2 0 0 2 2 2 2 2 2 2 2 2 0 0 0 2 2 2 2 2 2 2 2 2 2 2 2 2 2 2 2 2 2 2 2 2 2 2 2 2 2 2 2 2 2 2 2 2 2 2 2 2 2 2 3.12284933783e-14 0 2 2 2 2 2 2 2 2 2 2 2 2 2 2 2 2 2 2 2 2 2 2 2 2 2 2 2 2 2 2 2 2 2 2 2 2 2 2 2 2 2 2 2 2 2 2 2 2 2 2 2 2 2 2 2 2 2 2 2 2 2 2 2 2 2 2 2 2 2 2 2 2 2 2 3.12284933783e-14 0 2 2 2]
      | sbobj.Groups.TimeRange = [0 0.31]
  Call_Init1 : Outport
  DampgCmdBas : Outport  Tag=STV Outport  Port=2
  InertiaCmpVelCmd : Outport  Tag=STV Outport  Port=3
  AssiPahLimrActv : Outport  Tag=STV Outport  Port=4
  MotVelCrf : Outport  Tag=STV Outport  Port=5
  VehSpd : Outport  Tag=STV Outport  Port=6
  DampgCmdBasDi : Outport  Tag=STV Outport  Port=7
  MfgEnaSt : Outport  Tag=STV Outport  Port=8
  wires:
  FromWs/1 -> Demux/1
  Demux/1 -> Call_Init1/1
  Demux/2 -> DampgCmdBas/1
  Demux/3 -> InertiaCmpVelCmd/1
  Demux/4 -> AssiPahLimrActv/1
  Demux/5 -> MotVelCrf/1
  Demux/6 -> VehSpd/1
  Demux/7 -> DampgCmdBasDi/1
  Demux/8 -> MfgEnaSt/1

== system SF035A_DampgPahFwl/DampgPahFwl/CopyRight2 ==

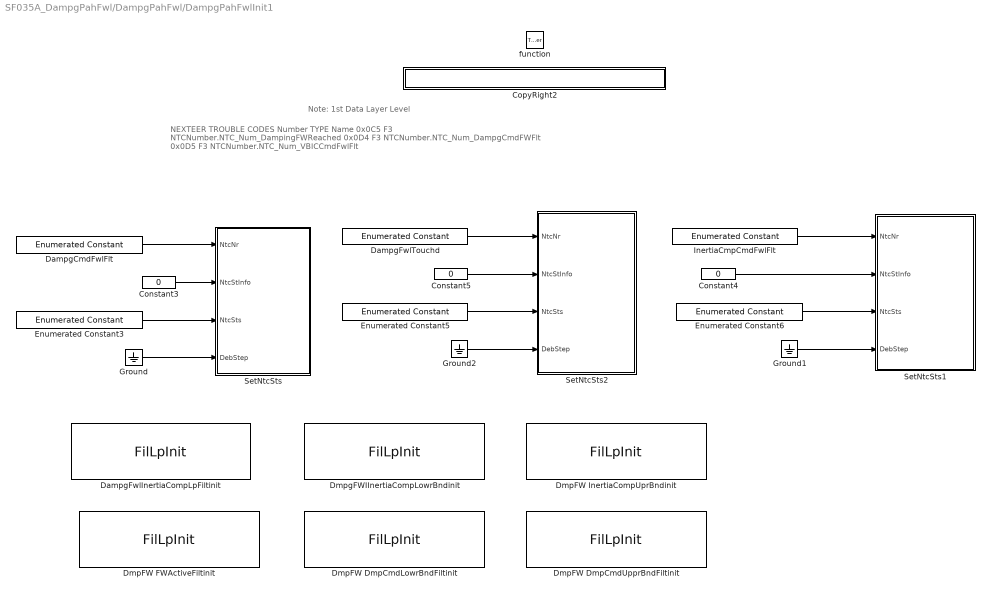
== system SF035A_DampgPahFwl/DampgPahFwl/DampgPahFwlInit1 ==
  note: Note: 1st Data Layer Level
  note: NEXTEER TROUBLE CODES
      | Number  TYPE   Name
      |
      |  0x0C5      F3      NTCNumber.NTC_Num_DampingFWReached
      |  0x0D4      F3      NTCNumber.NTC_Num_DampgCmdFWFlt
      |  0x0D5      F3      NTCNumber.NTC_Num_VBICCmdFwlFlt
  function : TriggerPort  TriggerType=function-call
  Constant3 : Constant  RequirementInfo={} %GIDa_2bcab23c_2e88_4dcf_a825_10b5d60e7fb9  Value=0  OutDataTypeStr=uint8
      settings: AttributesFormatString=%<OutDataTypeStr>
  Constant4 : Constant  RequirementInfo={} %GIDa_f6a70f41_fe71_4cee_8899_4f6519221115  Value=0  OutDataTypeStr=uint8
      settings: AttributesFormatString=%<OutDataTypeStr>
  Constant5 : Constant  RequirementInfo={} %GIDa_98e3dfc8_c11a_44db_a89c_49b318187b6d  Value=0  OutDataTypeStr=uint8
      settings: AttributesFormatString=%<OutDataTypeStr>
  CopyRight2 : Subsystem  Description=|  mask(Copyright Information){none=on}
      | Copyright info block.                                               
      |                                                                     
      | Place copyright information at the top of every subsystem in design.
      mask prompts: none "No parameters"
      mask help: Place copyright information at the top of every subsystem in design.
      mask Display:
      | NxtrConf = 'Nexteer Confidential';
      | 
      | sys = bdroot; %handle for the current model ("system")
      | first = get_param(sys,'Created');
      | first = first(end-3:end);  %year is last four digits
      | 
      | last = get_param(sys,'LastModifiedDate');
      | if isempty(last)
      |     last = datestr(now,'yyyy');
      | else
      |     last = last(end-3:end);
      | end
      | 
      | if strcmp(first,last)
      |     fprintf('%s -- Copyright %s Nexteer',NxtrConf,first)
      | else
      |     fprintf('%s -- %s%s- %s Nexteer',NxtrConf,char(169),first,last)
      | end
  DampgCmdFwlFlt : simulink/Sources/Enumerated Constant  OutDataTypeStr=Enum: NtcNr1  Value=NtcNr1.NTCNR_0X0D4  SampleTime=inf
  DampgFwlInertiaCompLpFiltinit : Fil/FilLpInit  Ic=0  Ts=ARCHGLBPRM_2MILLISEC_SEC_F32  Freq=DampgPahFwlInertiaCmpLpFilFrq  StVar=InertiaCmpLpFil
  DampgFwlTouchd : simulink/Sources/Enumerated Constant  OutDataTypeStr=Enum: NtcNr1  Value=NtcNr1.NTCNR_0X0C5  SampleTime=inf
  DmpFW DmpCmdLowrBndFiltinit : Fil/FilLpInit  Ic=0  Ts=ARCHGLBPRM_2MILLISEC_SEC_F32  Freq=DampgPahFwlDampgCmdLpFilFrq  StVar=DampgCmdLpFilLowrLim
  DmpFW DmpCmdUpprBndFiltinit : Fil/FilLpInit  Ic=0  Ts=ARCHGLBPRM_2MILLISEC_SEC_F32  Freq=DampgPahFwlDampgCmdLpFilFrq  StVar=DampgCmdLpFilUpprLim
  DmpFW FWActiveFiltinit : Fil/FilLpInit  Ic=0  Ts=ARCHGLBPRM_2MILLISEC_SEC_F32  Freq=DampgPahFwlActvFwlLpFilFrq  StVar=FwlActvLpFil
  DmpFW InertiaCompUprBndinit : Fil/FilLpInit  Ic=0  Ts=ARCHGLBPRM_2MILLISEC_SEC_F32  Freq=DampgPahFwlInertiaCmpLpFilFrq  StVar=InertiaCmpLpFilUpprLim
  DmpgFWIInertiaCompLowrBndinit : Fil/FilLpInit  Ic=0  Ts=ARCHGLBPRM_2MILLISEC_SEC_F32  Freq=DampgPahFwlInertiaCmpLpFilFrq  StVar=InertiaCmpLpFilLowrLim
  Enumerated Constant3 : simulink/Sources/Enumerated Constant  OutDataTypeStr=Enum: NtcSts1  Value=NtcSts1.NTCSTS_PASSD  SampleTime=inf
  Enumerated Constant5 : simulink/Sources/Enumerated Constant  OutDataTypeStr=Enum: NtcSts1  Value=NtcSts1.NTCSTS_PASSD  SampleTime=inf
  Enumerated Constant6 : simulink/Sources/Enumerated Constant  OutDataTypeStr=Enum: NtcSts1  Value=NtcSts1.NTCSTS_PASSD  SampleTime=inf
  Ground : Ground
  Ground1 : Ground
  Ground2 : Ground
  InertiaCmpCmdFwlFlt : simulink/Sources/Enumerated Constant  OutDataTypeStr=Enum: NtcNr1  Value=NtcNr1.NTCNR_0X0D5  SampleTime=inf
  SetNtcSts : Subsystem  mask(SetNTC){}
      mask help: SetNTC library block
  SetNtcSts1 : Subsystem  mask(SetNTC){}
      mask help: SetNTC library block
  SetNtcSts2 : Subsystem  mask(SetNTC){}
      mask help: SetNTC library block
  wires:
  Ground/1 -> SetNtcSts/4(DebStep)
  DampgCmdFwlFlt/1 -> SetNtcSts/1(NtcNr)
  Enumerated Constant3/1 -> SetNtcSts/3(NtcSts)
  Constant3/1 -> SetNtcSts/2(NtcStInfo)
  Ground2/1 -> SetNtcSts2/4(DebStep)
  DampgFwlTouchd/1 -> SetNtcSts2/1(NtcNr)
  Enumerated Constant5/1 -> SetNtcSts2/3(NtcSts)
  Constant5/1 -> SetNtcSts2/2(NtcStInfo)
  Ground1/1 -> SetNtcSts1/4(DebStep)
  InertiaCmpCmdFwlFlt/1 -> SetNtcSts1/1(NtcNr)
  Enumerated Constant6/1 -> SetNtcSts1/3(NtcSts)
  Constant4/1 -> SetNtcSts1/2(NtcStInfo)

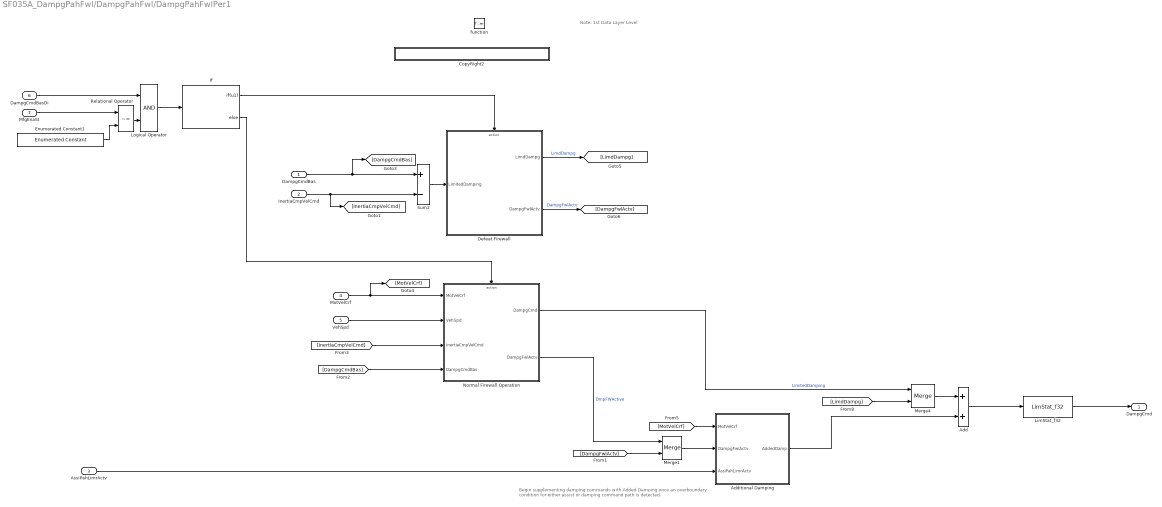
== system SF035A_DampgPahFwl/DampgPahFwl/DampgPahFwlPer1 ==
  note: Note: 1st Data Layer Level
  note: Begin supplementing damping commands with Added Damping once
      | an overboundary condition for either assist or damping command path is detected.
  DampgCmdBas : Inport
  InertiaCmpVelCmd : Inport  Port=2
  AssiPahLimrActv : Inport  Port=3
  MotVelCrf : Inport  Port=4
  VehSpd : Inport  Port=5
  DampgCmdBasDi : Inport  Port=6
  MfgEnaSt : Inport  Port=7
  function : TriggerPort  TriggerType=function-call
  Add : Sum
  Additional Damping : Subsystem
  CopyRight2 : Subsystem  Description=|  mask(Copyright Information){none=on}
      | Copyright info block.                                               
      |                                                                     
      | Place copyright information at the top of every subsystem in design.
      mask prompts: none "No parameters"
      mask help: Place copyright information at the top of every subsystem in design.
      mask Display:
      | NxtrConf = 'Nexteer Confidential';
      | 
      | sys = bdroot; %handle for the current model ("system")
      | first = get_param(sys,'Created');
      | first = first(end-3:end);  %year is last four digits
      | 
      | last = get_param(sys,'LastModifiedDate');
      | if isempty(last)
      |     last = datestr(now,'yyyy');
      | else
      |     last = last(end-3:end);
      | end
      | 
      | if strcmp(first,last)
      |     fprintf('%s -- Copyright %s Nexteer',NxtrConf,first)
      | else
      |     fprintf('%s -- %s%s- %s Nexteer',NxtrConf,char(169),first,last)
      | end
  Defeat Firewall : Subsystem  TreatAsAtomicUnit=on
  Enumerated Constant1 : simulink/Sources/Enumerated Constant  RequirementInfo={} %GIDa_469b8d3d_ae37_4908_9895_634ba76d4e42  OutDataTypeStr=Enum: MfgEnaSt1  Value=MfgEnaSt1.MFGENAST_PRDNMOD  SampleTime=inf
  If : If  IfExpression=u1
  LimStat_f32 : NxtrLim/LimStat_f32  LoLim=SYSGLBPRM_MOTTQCMDLOLIM_MOTNWTMTR_F32  HiLim=SYSGLBPRM_MOTTQCMDHILIM_MOTNWTMTR_F32
      settings: AttributesFormatString=|
      | Low Limit: %<LoLim>
      | High Limit:%<HiLim>
  Logical Operator : Logic  AllPortsSameDT=off  OutDataTypeStr=boolean
  Merge1 : Merge
  Merge4 : Merge
  Normal Firewall Operation : Subsystem  TreatAsAtomicUnit=on
  Relational Operator : RelationalOperator  Operator=~=  OutDataTypeStr=boolean
  Sum2 : Sum  Inputs=+-  SaturateOnIntegerOverflow=on  InputSameDT=on  OutDataTypeStr=Inherit: Same as first input
  DampgCmd : Outport
  wires:
  VehSpd/1 -> Normal Firewall Operation/2(VehSpd)
  MotVelCrf/1 -> [MotVelCrf], Normal Firewall Operation/1(MotVelCrf)
  If/2 -> Normal Firewall Operation/Action
  If/1 -> Defeat Firewall/Action
  InertiaCmpVelCmd/1 -> Sum2/2, [InertiaCmpVelCmd]
  Sum2/1 -> Defeat Firewall/1(LimitedDamping)
  LimStat_f32/1 -> DampgCmd/1
  Additional Damping/1(AddedDamp) -> Add/2
  Merge4/1 -> Add/1
  Merge1/1 -> Additional Damping/2(DampgFwlActv)
  [MotVelCrf] -> Additional Damping/1(MotVelCrf)
  AssiPahLimrActv/1 -> Additional Damping/3(AssiPahLimrActv)
  Logical Operator/1 -> If/1
  DampgCmdBasDi/1 -> Logical Operator/1
  Relational Operator/1 -> Logical Operator/2
  Defeat Firewall/1(LimdDampg) -> [LimdDampg]  "LimdDampg"
  Defeat Firewall/2(DampgFwlActv) -> [DampgFwlActv]  "DampgFwlActv"
  Normal Firewall Operation/2(DampgFwlActv) -> Merge1/1  "DmpFWActive"
  [DampgFwlActv] -> Merge1/2
  Normal Firewall Operation/1(DampgCmd) -> Merge4/1  "LimitedDamping"
  [LimdDampg] -> Merge4/2
  DampgCmdBas/1 -> Sum2/1, [DampgCmdBas]
  [InertiaCmpVelCmd] -> Normal Firewall Operation/3(InertiaCmpVelCmd)
  [DampgCmdBas] -> Normal Firewall Operation/4(DampgCmdBas)
  Add/1 -> LimStat_f32/1
  Enumerated Constant1/1 -> Relational Operator/2
  MfgEnaSt/1 -> Relational Operator/1

== system SF035A_DampgPahFwl/Init Trigger/CopyRight2 ==

== system SF035A_DampgPahFwl/DampgPahFwl/DampgPahFwlInit1/CopyRight2 ==

== system SF035A_DampgPahFwl/DampgPahFwl/DampgPahFwlInit1/SetNtcSts ==
  NtcNr : Inport
  NtcStInfo : Inport  Port=2
  NtcSts : Inport  Port=3
  DebStep : Inport  Port=4
  SetNtcSts : Subsystem  RequirementInfo={} %GIDa_2eb96cd9_148a_4ca2_a8f4_805dd7868ab6  TreatAsAtomicUnit=on
      settings: RTWSystemCode=Inline
  wires:
  NtcNr/1 -> SetNtcSts/1(NtcNr)  "NtcNr"
  NtcSts/1 -> SetNtcSts/3(NtcSts)
  DebStep/1 -> SetNtcSts/4(DebStep)
  NtcStInfo/1 -> SetNtcSts/2(NtcStInfo)

== system SF035A_DampgPahFwl/DampgPahFwl/DampgPahFwlInit1/SetNtcSts1 ==
  NtcNr : Inport
  NtcStInfo : Inport  Port=2
  NtcSts : Inport  Port=3
  DebStep : Inport  Port=4
  SetNtcSts : Subsystem  RequirementInfo={} %GIDa_d572260a_e585_40fd_a4d8_7370a643af8d  TreatAsAtomicUnit=on
      settings: RTWSystemCode=Inline
  wires:
  NtcNr/1 -> SetNtcSts/1(NtcNr)  "NtcNr"
  NtcSts/1 -> SetNtcSts/3(NtcSts)
  DebStep/1 -> SetNtcSts/4(DebStep)
  NtcStInfo/1 -> SetNtcSts/2(NtcStInfo)

== system SF035A_DampgPahFwl/DampgPahFwl/DampgPahFwlInit1/SetNtcSts2 ==
  NtcNr : Inport
  NtcStInfo : Inport  Port=2
  NtcSts : Inport  Port=3
  DebStep : Inport  Port=4
  SetNtcSts : Subsystem  RequirementInfo={} %GIDa_db1daf49_ad74_490e_acfd_468080e007a9  TreatAsAtomicUnit=on
      settings: RTWSystemCode=Inline
  wires:
  NtcNr/1 -> SetNtcSts/1(NtcNr)  "NtcNr"
  NtcSts/1 -> SetNtcSts/3(NtcSts)
  DebStep/1 -> SetNtcSts/4(DebStep)
  NtcStInfo/1 -> SetNtcSts/2(NtcStInfo)

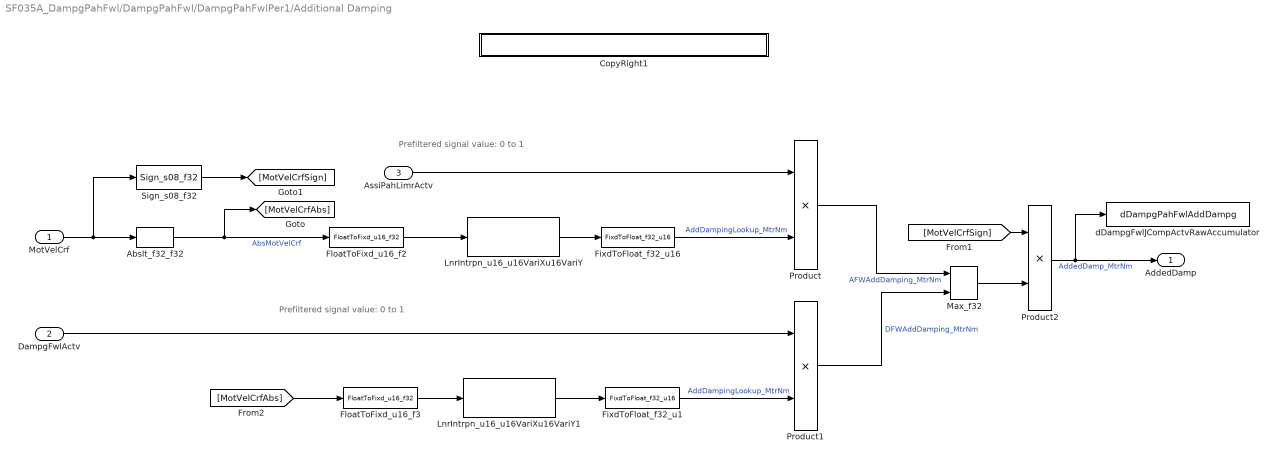
== system SF035A_DampgPahFwl/DampgPahFwl/DampgPahFwlPer1/Additional Damping ==
  note: Prefiltered signal
      | value:  0 to 1
  note: Prefiltered signal
      | value:  0 to 1
  MotVelCrf : Inport
  DampgFwlActv : Inport  Port=2
  AssiPahLimrActv : Inport  Port=3
  Abslt_f32_f32 : NxtrAbslt/Abslt_f32_f32  SFunctionSpec=single y1 = Abslt_f32_f32(single u1)
      settings: AttributesFormatString=%<Name>
  CopyRight1 : Subsystem  Description=|  mask(Copyright Information){none=on}
      | Copyright info block.                                               
      |                                                                     
      | Place copyright information at the top of every subsystem in design.
      mask prompts: none "No parameters"
      mask help: Place copyright information at the top of every subsystem in design.
      mask Display:
      | NxtrConf = 'Nexteer Confidential';
      | 
      | sys = bdroot; %handle for the current model ("system")
      | first = get_param(sys,'Created');
      | first = first(end-3:end);  %year is last four digits
      | 
      | last = get_param(sys,'LastModifiedDate');
      | if isempty(last)
      |     last = datestr(now,'yyyy');
      | else
      |     last = last(end-3:end);
      | end
      | 
      | if strcmp(first,last)
      |     fprintf('%s -- Copyright %s Nexteer',NxtrConf,first)
      | else
      |     fprintf('%s -- %s%s- %s Nexteer',NxtrConf,char(169),first,last)
      | end
  FixdToFloat_f32_u1 : FixdToFloat/FixdToFloat_f32_u16  Param1=11
  FixdToFloat_f32_u16 : FixdToFloat/FixdToFloat_f32_u16  Param1=11
  FloatToFixd_u16_f2 : FloatToFixd/FloatToFixd_u16_f32  Param1=5
  FloatToFixd_u16_f3 : FloatToFixd/FloatToFixd_u16_f32  Param1=5
  LnrIntrpn_u16_u16VariXu16VariY : LnrIntrpn/LnrIntrpn_u16_u16VariXu16VariY  XTbl=DampgPahFwlAssiAddlDampgX  YTbl=DampgPahFwlAssiAddlDampgY
      settings: AttributesFormatString=Lnr ( u16VariX , u16VariY )
  LnrIntrpn_u16_u16VariXu16VariY1 : LnrIntrpn/LnrIntrpn_u16_u16VariXu16VariY  XTbl=DampgPahFwlDampgCmdAddlDampgX  YTbl=DampgPahFwlDampgCmdAddlDampgY
      settings: AttributesFormatString=Lnr ( u16VariX , u16VariY )
  Max_f32 : NxtrMax/Max_f32  SFunctionSpec=single y1 = Max_f32(single u1, single u2)
      settings: AttributesFormatString=%<Name>
  Product : Product  RndMeth=Zero
  Product1 : Product  RndMeth=Zero
  Product2 : Product  RndMeth=Zero
  Sign_s08_f32 : NxtrSign/Sign_s08_f32  SFunctionSpec=int8 y1 = Sign_s08_f32(single u1)
  dDampgFwlJCompActvRawAccumulator : DataStoreWrite  DataStoreName=dDampgPahFwlAddDampg
  AddedDamp : Outport
  wires:
  MotVelCrf/1 -> Abslt_f32_f32/1, Sign_s08_f32/1
  FixdToFloat_f32_u16/1 -> Product/2  "AddDampingLookup_MtrNm"
  AssiPahLimrActv/1 -> Product/1
  Abslt_f32_f32/1 -> FloatToFixd_u16_f2/1, [MotVelCrfAbs]  "AbsMotVelCrf"
  Sign_s08_f32/1 -> [MotVelCrfSign]
  FixdToFloat_f32_u1/1 -> Product1/2  "AddDampingLookup_MtrNm"
  DampgFwlActv/1 -> Product1/1
  [MotVelCrfAbs] -> FloatToFixd_u16_f3/1
  Product/1 -> Max_f32/1  "AFWAddDamping_MtrNm"
  Product1/1 -> Max_f32/2  "DFWAddDamping_MtrNm"
  [MotVelCrfSign] -> Product2/1
  Max_f32/1 -> Product2/2
  Product2/1 -> dDampgFwlJCompActvRawAccumulator/1, AddedDamp/1  "AddedDamp_MtrNm"
  FloatToFixd_u16_f2/1 -> LnrIntrpn_u16_u16VariXu16VariY/1
  LnrIntrpn_u16_u16VariXu16VariY/1 -> FixdToFloat_f32_u16/1
  FloatToFixd_u16_f3/1 -> LnrIntrpn_u16_u16VariXu16VariY1/1
  LnrIntrpn_u16_u16VariXu16VariY1/1 -> FixdToFloat_f32_u1/1

== system SF035A_DampgPahFwl/DampgPahFwl/DampgPahFwlPer1/CopyRight2 ==

== system SF035A_DampgPahFwl/DampgPahFwl/DampgPahFwlPer1/Defeat Firewall ==
  LimitedDamping : Inport
  Action Port : ActionPort  ActionType=then
  Constant4 : Constant  Value=0  OutDataTypeStr=single
      settings: AttributesFormatString=%<OutDataTypeStr>
  CopyRight2 : Subsystem  Description=|  mask(Copyright Information){none=on}
      | Copyright info block.                                               
      |                                                                     
      | Place copyright information at the top of every subsystem in design.
      mask prompts: none "No parameters"
      mask help: Place copyright information at the top of every subsystem in design.
      mask Display:
      | NxtrConf = 'Nexteer Confidential';
      | 
      | sys = bdroot; %handle for the current model ("system")
      | first = get_param(sys,'Created');
      | first = first(end-3:end);  %year is last four digits
      | 
      | last = get_param(sys,'LastModifiedDate');
      | if isempty(last)
      |     last = datestr(now,'yyyy');
      | else
      |     last = last(end-3:end);
      | end
      | 
      | if strcmp(first,last)
      |     fprintf('%s -- Copyright %s Nexteer',NxtrConf,first)
      | else
      |     fprintf('%s -- %s%s- %s Nexteer',NxtrConf,char(169),first,last)
      | end
  LimdDampg : Outport
  DampgFwlActv : Outport  Port=2
  wires:
  LimitedDamping/1 -> LimdDampg/1
  Constant4/1 -> DampgFwlActv/1

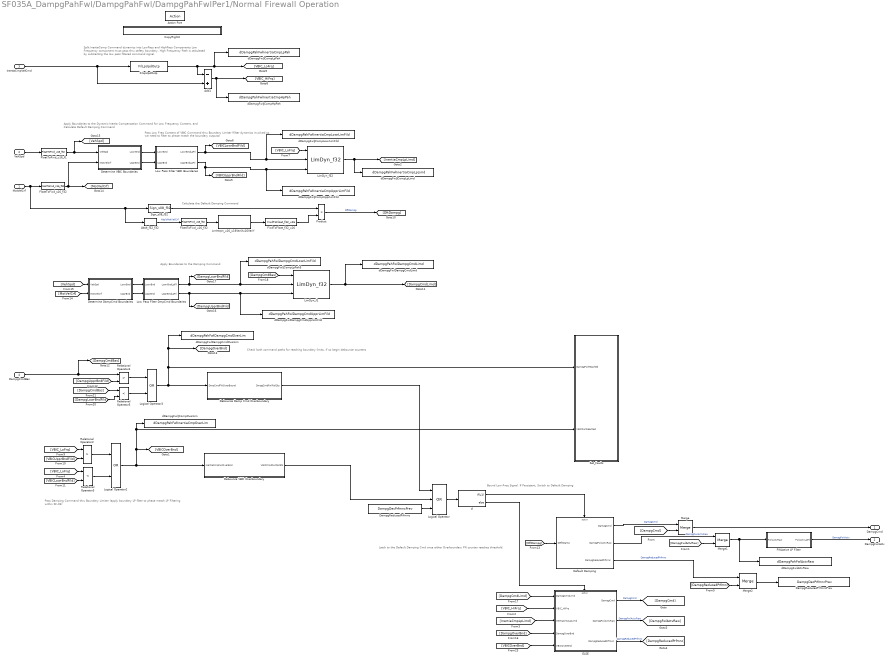
== system SF035A_DampgPahFwl/DampgPahFwl/DampgPahFwlPer1/Normal Firewall Operation ==
  note: Bound Low-Freq Signal. If Persistent, Switch to Default Damping
  note: Check both command paths for reaching boundary limits, if so begin debounce counters
  note: Split InertiaComp Command dynamics into LowPass and HighPass Components
      | Low Frequency component must pass thru safety boundary.  High Frequency
      | Path is calculated by subtracting the low pass filtered command signal.
  note: Pass Damping Command thru Boundary Limiter (apply boundary LP filter to phase match LP Filtering within SF-03)
  note: Pass Low Freq Content of VBIC Command thru Boundary Limiter
      | (filter dynamics involved so we need to filter to phase match the boundary outputs)
  note: Apply Boundaries to the Dynamic Inertia Compensation Command for Low Frequency Content, and Calculate Default Damping Command
  note: Calculate the Default Damping Command
  note: Latch to the Default Damping Cmd once either Overboundary PN counter reaches threshold.
  note: Apply Boundaries to the Damping Command
  MotVelCrf : Inport
  VehSpd : Inport  Port=2
  InertiaCmpVelCmd : Inport  Port=3
  DampgCmdBas : Inport  Port=4
  Action Port : ActionPort  ActionType=else
  Abslt_f32_f32 : NxtrAbslt/Abslt_f32_f32  SFunctionSpec=single y1 = Abslt_f32_f32(single u1)
      settings: AttributesFormatString=%<Name>
  Add1 : Sum  Inputs=-+
  CopyRight2 : Subsystem  Description=|  mask(Copyright Information){none=on}
      | Copyright info block.                                               
      |                                                                     
      | Place copyright information at the top of every subsystem in design.
      mask prompts: none "No parameters"
      mask help: Place copyright information at the top of every subsystem in design.
      mask Display:
      | NxtrConf = 'Nexteer Confidential';
      | 
      | sys = bdroot; %handle for the current model ("system")
      | first = get_param(sys,'Created');
      | first = first(end-3:end);  %year is last four digits
      | 
      | last = get_param(sys,'LastModifiedDate');
      | if isempty(last)
      |     last = datestr(now,'yyyy');
      | else
      |     last = last(end-3:end);
      | end
      | 
      | if strcmp(first,last)
      |     fprintf('%s -- Copyright %s Nexteer',NxtrConf,first)
      | else
      |     fprintf('%s -- %s%s- %s Nexteer',NxtrConf,char(169),first,last)
      | end
  DampgReducedPrfmnc : DataStoreRead  DataStoreName=DampgDecPrfmncPrev
  DampgReducedPrfmncPrev : DataStoreWrite  DataStoreName=DampgDecPrfmncPrev
  Debounce Damp Cmd Overboundary : Subsystem
  Debounce VBIC Overboundary : Subsystem
  Default Damping : Subsystem  TreatAsAtomicUnit=on
  Determine DampCmd Boundaries : Subsystem
  Determine VBIC Boundaries : Subsystem
  ELSE : Subsystem  TreatAsAtomicUnit=on
  FWActive LP Filter : Subsystem
  FilLpUpdOutp : Fil/FilLpUpdOutp  StVar=InertiaCmpLpFil
      settings: AttributesFormatString=StVar: %<StVar>
  FixdToFloat_f32_u16 : FixdToFloat/FixdToFloat_f32_u16  Param1=11
  FloatToFixd_s16_f32 : FloatToFixd/FloatToFixd_s16_f32  Param1=4
  FloatToFixd_u16_f1 : FloatToFixd/FloatToFixd_u16_f32  Param1=7
  FloatToFixd_u16_f32 : FloatToFixd/FloatToFixd_u16_f32  Param1=5
  If : If  IfExpression=u1
  LimDyn_f1 : NxtrLim/LimDyn_f32
  LimDyn_f32 : NxtrLim/LimDyn_f32
  LnrIntrpn_u16_u16VariXu16VariY : LnrIntrpn/LnrIntrpn_u16_u16VariXu16VariY  XTbl=DampgPahFwlDftDampgX  YTbl=DampgPahFwlDftDampgY
      settings: AttributesFormatString=Lnr ( u16VariX , u16VariY )
  Logical Operator : Logic  Operator=OR  Inputs=3  AllPortsSameDT=off  OutDataTypeStr=boolean
  Logical Operator2 : Logic  Operator=OR  AllPortsSameDT=off  OutDataTypeStr=boolean
  Logical Operator3 : Logic  Operator=OR  AllPortsSameDT=off  OutDataTypeStr=boolean
  Low Pass Filter DmpCmd Boundaries : Subsystem
  Low Pass Filter VBIC Boundaries : Subsystem
  Merge : Merge
  Merge1 : Merge
  Merge2 : Merge
  Product : Product  RndMeth=Zero
  Relational Operator2 : RelationalOperator  Operator=>  OutDataTypeStr=boolean
  Relational Operator3 : RelationalOperator  Operator=<  OutDataTypeStr=boolean
  Relational Operator4 : RelationalOperator  Operator=>  OutDataTypeStr=boolean
  Relational Operator5 : RelationalOperator  Operator=<  OutDataTypeStr=boolean
  Set_Faults : Subsystem
  Sign_s08_f32 : NxtrSign/Sign_s08_f32  SFunctionSpec=int8 y1 = Sign_s08_f32(single u1)
  dDampgFwlActvRaw : DataStoreWrite  DataStoreName=dDampgPahFwlActvRaw
  dDampgFwlDampgCmdLimd : DataStoreWrite  DataStoreName=dDampgPahFwlDampgCmdLimd
  dDampgFwlDampgCmdOverLim : DataStoreWrite  DataStoreName=dDampgPahFwlDampgCmdOverLim
  dDampgFwlDampgCmdUpprLimFild : DataStoreWrite  DataStoreName=dDampgPahFwlDampgCmdUpprLimFild
  dDampgFwlJCompHpPah : DataStoreWrite  DataStoreName=dDampgPahFwlInertiaCmpHpPah
  dDampgFwlJCompLowrLimFild : DataStoreWrite  DataStoreName=dDampgPahFwlInertiaCmpLowrLimFild
  dDampgFwlJCompLpLimd : DataStoreWrite  DataStoreName=dDampgPahFwlInertiaCmpLpLimd
  dDampgFwlJCompLpPah : DataStoreWrite  DataStoreName=dDampgPahFwlInertiaCmpLpPah
  dDampgFwlJCompLpPah5 : DataStoreWrite  DataStoreName=dDampgPahFwlDampgCmdLowrLimFild
  dDampgFwlJCompOverLim : DataStoreWrite  DataStoreName=dDampgPahFwlInertiaCmpOverLim
  dDampgFwlJCompUpprLimFild : DataStoreWrite  DataStoreName=dDampgPahFwlInertiaCmpUpprLimFild
  DampgCmd : Outport
  DampgFwlActv : Outport  Tag=0x0C6  Port=2
  wires:
  FWActive LP Filter/1(FwlActvLpFil) -> DampgFwlActv/1  "DampgFwlActv"
  [VBIC_LoFrq] -> LimDyn_f32/1
  LimDyn_f32/1 -> dDampgFwlJCompLpLimd/1, [InertiaCmpLpLimd]
  [VBIC_HiFrq] -> ELSE/2(VBIC_HiFrq)
  Logical Operator/1 -> If/1
  [VBIC_LoFrq] -> Relational Operator2/1
  [VBIC_LoFrq] -> Relational Operator3/1
  Relational Operator2/1 -> Logical Operator2/1
  Relational Operator3/1 -> Logical Operator2/2
  [VBICUpprBndFild] -> Relational Operator2/2
  [VBICLowrBndFild] -> Relational Operator3/2
  If/1 -> Default Damping/Action
  If/2 -> ELSE/Action
  Product/1 -> [DftDampg]  "DftDampg"
  [DftDampg] -> Default Damping/1(DefltDamp)
  Default Damping/1(DampgCmd) -> Merge/1  "DampgCmd"
  Default Damping/2(DampgFwlActvRaw) -> Merge1/1  "DampgFwlActvRaw"
  Default Damping/3(DampgReducedPrfmnc) -> Merge2/1  "DampgReducedPrfmnc"
  Merge1/1 -> dDampgFwlActvRaw/1, FWActive LP Filter/1(FwlActvRaw)
  Merge2/1 -> DampgReducedPrfmncPrev/1
  InertiaCmpVelCmd/1 -> FilLpUpdOutp/1, Add1/2
  FilLpUpdOutp/1 -> dDampgFwlJCompLpPah/1, [VBIC_LoFrq], Add1/1
  [DampgOverBnd] -> ELSE/4(DampgOverBnd)
  DampgCmdBas/1 -> [DampgCmdBas], Relational Operator4/1
  [DampgCmdBas] -> Relational Operator5/1
  Relational Operator4/1 -> Logical Operator3/1
  Relational Operator5/1 -> Logical Operator3/2
  [DampgUpprBndFild] -> Relational Operator4/2
  [DampgLowrBndFild] -> Relational Operator5/2
  Logical Operator3/1 -> Set_Faults/1(DampgFwlReached), dDampgFwlDampgCmdOverLim/1, [DampgOverBnd], Debounce Damp Cmd Overboundary/1(DmpCmdFWOverBound)
  [VBICOverBnd] -> ELSE/5(VBICOverBnd)
  Merge/1 -> DampgCmd/1
  Sign_s08_f32/1 -> Product/1
  MotVelCrf/1 -> Abslt_f32_f32/1, Sign_s08_f32/1, FloatToFixd_s16_f32/1
  VehSpd/1 -> FloatToFixd_u16_f1/1
  Add1/1 -> dDampgFwlJCompHpPah/1, [VBIC_HiFrq]
  Determine VBIC Boundaries/1(LowrBnd) -> Low Pass Filter VBIC Boundaries/1(LowrBnd)
  Determine VBIC Boundaries/2(UpprBnd) -> Low Pass Filter VBIC Boundaries/2(UpprBnd)
  Low Pass Filter VBIC Boundaries/1(LowrBndLpFil) -> [VBICLowrBndFild], dDampgFwlJCompLowrLimFild/1, LimDyn_f32/2
  Low Pass Filter VBIC Boundaries/2(UpprBndLpFil) -> [VBICUpprBndFild], dDampgFwlJCompUpprLimFild/1, LimDyn_f32/3
  FloatToFixd_u16_f32/1 -> LnrIntrpn_u16_u16VariXu16VariY/1
  LnrIntrpn_u16_u16VariXu16VariY/1 -> FixdToFloat_f32_u16/1
  FixdToFloat_f32_u16/1 -> Product/2
  Abslt_f32_f32/1 -> FloatToFixd_u16_f32/1  "AbsltMotVelCrf"
  [MotVelCrf] -> Determine DampCmd Boundaries/2(MotVelCrf)
  [VehSpd] -> Determine DampCmd Boundaries/1(VehSpd)
  LimDyn_f1/1 -> [DampgCmdLimd], dDampgFwlDampgCmdLimd/1
  [DampgCmdBas] -> LimDyn_f1/1
  Determine DampCmd Boundaries/1(LowrBnd) -> Low Pass Filter DmpCmd Boundaries/1(LowrBnd)
  Determine DampCmd Boundaries/2(UpprBnd) -> Low Pass Filter DmpCmd Boundaries/2(UpprBnd)
  Low Pass Filter DmpCmd Boundaries/1(LowrBndLpFil) -> [DampgLowrBndFild], dDampgFwlJCompLpPah5/1, LimDyn_f1/2
  Low Pass Filter DmpCmd Boundaries/2(UpprBndLpFil) -> [DampgUpprBndFild], dDampgFwlDampgCmdUpprLimFild/1, LimDyn_f1/3
  [DampgCmdLimd] -> ELSE/1(DampgCmdLimd)
  DampgReducedPrfmnc/1 -> Logical Operator/3
  Logical Operator2/1 -> Set_Faults/2(VBICFwlReached), dDampgFwlJCompOverLim/1, [VBICOverBnd], Debounce VBIC Overboundary/1(InertiaCmpFwlOverBnd)
  Debounce Damp Cmd Overboundary/1(DmpgCmdFwlFailSts) -> Logical Operator/1
  Debounce VBIC Overboundary/1(VBICCmdFwlFailSts) -> Logical Operator/2
  FloatToFixd_u16_f1/1 -> [VehSpd], Determine VBIC Boundaries/1(VehSpd)
  FloatToFixd_s16_f32/1 -> [MotVelCrf], Determine VBIC Boundaries/2("MotVelCrf ")
  ELSE/1(DampgCmd) -> [DampgCmd]  "DampgCmd"
  [DampgCmd] -> Merge/2
  ELSE/2(DampgFwlActvRaw) -> [DampgFwlActvRaw]  "DampgFwlActvRaw"
  [DampgFwlActvRaw] -> Merge1/2
  ELSE/3(DampgReducedPrfmnc) -> [DampgReducedPrfmnc]  "DampgReducedPrfmnc"
  [DampgReducedPrfmnc] -> Merge2/2
  [InertiaCmpLpLimd] -> ELSE/3(InertiaCmpLpLimd)

== system SF035A_DampgPahFwl/DampgPahFwl/DampgPahFwlInit1/SetNtcSts/SetNtcSts ==
  note: Note:
      |
      | - "ISO Fault Debounce Design" Simulink block intent to use here for Simulation purpose only. Do not Code this block
  NtcNr : Inport
  NtcStInfo : Inport  Port=2
  NtcSts : Inport  Port=3
  DebStep : Inport  Port=4
  CopyRight2 : Subsystem  Description=|  mask(Copyright Information){none=on}
      | Copyright info block.                                               
      |                                                                     
      | Place copyright information at the top of every subsystem in design.
      mask prompts: none "No parameters"
      mask help: Place copyright information at the top of every subsystem in design.
      mask Display:
      | NxtrConf = 'Nexteer Confidential';
      | 
      | sys = bdroot; %handle for the current model ("system")
      | first = get_param(sys,'Created');
      | first = first(end-3:end);  %year is last four digits
      | 
      | last = get_param(sys,'LastModifiedDate');
      | if isempty(last)
      |     last = datestr(now,'yyyy');
      | else
      |     last = last(end-3:end);
      | end
      | 
      | if strcmp(first,last)
      |     fprintf('%s -- Copyright %s Nexteer',NxtrConf,first)
      | else
      |     fprintf('%s -- %s%s- %s Nexteer',NxtrConf,char(169),first,last)
      | end
  Data Type Conversion : DataTypeConversion  OutDataTypeStr=Enum: SigQlfr1
  Ground : Ground
  ISO Fault Debounce Design : Stateflow chart  TreatAsAtomicUnit=on
      settings: AttributesFormatString=|
      | Simulation Purpose Only.
      | Do Not Code this block
      | Diagnostic Manager Owns this requirement
  Ntc0x0D4Qlfr : DataStoreWrite  DataStoreName=Ntc0X0D4Qlfr
  Terminator : Terminator
  Terminator1 : Terminator
  wires:
  NtcStInfo/1 -> Terminator1/1
  NtcNr/1 -> Terminator/1
  NtcSts/1 -> ISO Fault Debounce Design/1(NtcSts)
  DebStep/1 -> ISO Fault Debounce Design/2(DebStep)
  ISO Fault Debounce Design/1(Qualifier) -> Data Type Conversion/1
  Ground/1 -> ISO Fault Debounce Design/3(SvcClr)
  Data Type Conversion/1 -> Ntc0x0D4Qlfr/1

== system SF035A_DampgPahFwl/DampgPahFwl/DampgPahFwlInit1/SetNtcSts1/SetNtcSts ==
  note: Note:
      |
      | - "ISO Fault Debounce Design" Simulink block intent to use here for Simulation purpose only. Do not Code this block
  NtcNr : Inport
  NtcStInfo : Inport  Port=2
  NtcSts : Inport  Port=3
  DebStep : Inport  Port=4
  CopyRight2 : Subsystem  Description=|  mask(Copyright Information){none=on}
      | Copyright info block.                                               
      |                                                                     
      | Place copyright information at the top of every subsystem in design.
      mask prompts: none "No parameters"
      mask help: Place copyright information at the top of every subsystem in design.
      mask Display:
      | NxtrConf = 'Nexteer Confidential';
      | 
      | sys = bdroot; %handle for the current model ("system")
      | first = get_param(sys,'Created');
      | first = first(end-3:end);  %year is last four digits
      | 
      | last = get_param(sys,'LastModifiedDate');
      | if isempty(last)
      |     last = datestr(now,'yyyy');
      | else
      |     last = last(end-3:end);
      | end
      | 
      | if strcmp(first,last)
      |     fprintf('%s -- Copyright %s Nexteer',NxtrConf,first)
      | else
      |     fprintf('%s -- %s%s- %s Nexteer',NxtrConf,char(169),first,last)
      | end
  Data Type Conversion : DataTypeConversion  OutDataTypeStr=Enum: SigQlfr1
  Ground : Ground
  ISO Fault Debounce Design : Stateflow chart  TreatAsAtomicUnit=on
      settings: AttributesFormatString=|
      | Simulation Purpose Only.
      | Do Not Code this block
      | Diagnostic Manager Owns this requirement
  Ntc0X0D4Qlfr : DataStoreWrite  DataStoreName=Ntc0X0D5Qlfr
  Terminator : Terminator
  Terminator1 : Terminator
  wires:
  NtcStInfo/1 -> Terminator1/1
  NtcNr/1 -> Terminator/1
  NtcSts/1 -> ISO Fault Debounce Design/1(NtcSts)
  DebStep/1 -> ISO Fault Debounce Design/2(DebStep)
  ISO Fault Debounce Design/1(Qualifier) -> Data Type Conversion/1
  Ground/1 -> ISO Fault Debounce Design/3(SvcClr)
  Data Type Conversion/1 -> Ntc0X0D4Qlfr/1

== system SF035A_DampgPahFwl/DampgPahFwl/DampgPahFwlInit1/SetNtcSts2/SetNtcSts ==
  note: Note:
      |
      | - "ISO Fault Debounce Design" Simulink block intent to use here for Simulation purpose only. Do not Code this block
  NtcNr : Inport
  NtcStInfo : Inport  Port=2
  NtcSts : Inport  Port=3
  DebStep : Inport  Port=4
  CopyRight2 : Subsystem  Description=|  mask(Copyright Information){none=on}
      | Copyright info block.                                               
      |                                                                     
      | Place copyright information at the top of every subsystem in design.
      mask prompts: none "No parameters"
      mask help: Place copyright information at the top of every subsystem in design.
      mask Display:
      | NxtrConf = 'Nexteer Confidential';
      | 
      | sys = bdroot; %handle for the current model ("system")
      | first = get_param(sys,'Created');
      | first = first(end-3:end);  %year is last four digits
      | 
      | last = get_param(sys,'LastModifiedDate');
      | if isempty(last)
      |     last = datestr(now,'yyyy');
      | else
      |     last = last(end-3:end);
      | end
      | 
      | if strcmp(first,last)
      |     fprintf('%s -- Copyright %s Nexteer',NxtrConf,first)
      | else
      |     fprintf('%s -- %s%s- %s Nexteer',NxtrConf,char(169),first,last)
      | end
  Data Type Conversion : DataTypeConversion  OutDataTypeStr=Enum: SigQlfr1
  Ground : Ground
  ISO Fault Debounce Design : Stateflow chart  TreatAsAtomicUnit=on
      settings: AttributesFormatString=|
      | Simulation Purpose Only.
      | Do Not Code this block
      | Diagnostic Manager Owns this requirement
  Ntc0x0C5Qlfr : DataStoreWrite  DataStoreName=Ntc0X0C5Qlfr
  Terminator : Terminator
  Terminator1 : Terminator
  wires:
  NtcStInfo/1 -> Terminator1/1
  NtcNr/1 -> Terminator/1
  NtcSts/1 -> ISO Fault Debounce Design/1(NtcSts)
  DebStep/1 -> ISO Fault Debounce Design/2(DebStep)
  ISO Fault Debounce Design/1(Qualifier) -> Data Type Conversion/1
  Ground/1 -> ISO Fault Debounce Design/3(SvcClr)
  Data Type Conversion/1 -> Ntc0x0C5Qlfr/1

== system SF035A_DampgPahFwl/DampgPahFwl/DampgPahFwlPer1/Additional Damping/CopyRight1 ==

== system SF035A_DampgPahFwl/DampgPahFwl/DampgPahFwlPer1/Defeat Firewall/CopyRight2 ==

== system SF035A_DampgPahFwl/DampgPahFwl/DampgPahFwlPer1/Normal Firewall Operation/CopyRight2 ==
